simulink model "MOD5"  (R2017a)
settings: Solver=FixedStepAuto  StartTime=0.0  StopTime=10  FixedStep=1/160000  RelTol=1e-3
undefined symbols (not defined in the file): H
libraries: dspmlti4 x4
settings Model: Creator=bhannigan  LastModifiedBy=bhannigan

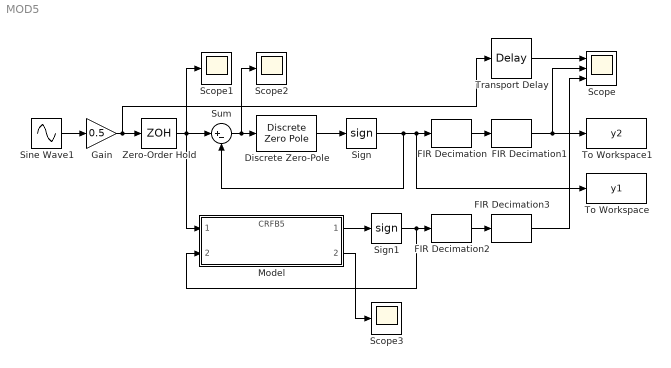
== system MOD5 ==
  Discrete Zero-Pole : DiscreteZeroPole  Zeros=H.Z{1}  Poles=H.P{1}  Gain=H.K  SampleTime=-1
  FIR Decimation{,1..3} (4 alike) : dspmlti4/FIR Decimation  FilterSource=Dialog parameters  h=fir1(31,1/64)  D=8  filtStruct=Direct form  FilterObject=FDECIM  framing=Allow multirate processing  inputOffset=0  outputBufInitCond=0  roundingMode=Floor  overflowMode=off  firstCoeffDataTypeStr=Inherit: Same word length as input  firstCoeffMin=[]  firstCoeffMax=[]  firstCoeffLastDataTypeStr=Inherit: Same word length as input  outputDataTypeStr=Inherit: Same as accumulator  outputMin=[]  outputMax=[]  outputLastDataTypeStr=Inherit: Same as accumulator
  Gain : Gain  Gain=0.5
  Model : ModelReference  ModelNameDialog=CRFB5  SimulationMode=Normal  ModelReferenceVersion=1.15
  Scope : Scope  NumInputPorts=3
  Scope1 : Scope
  Scope2 : Scope
  Scope3 : Scope
  Sign : Signum
  Sign1 : Signum
  Sine Wave1 : Sin  Frequency=2*pi*100  SampleTime=0
  Sum : Sum  Inputs=|+-
  To Workspace : ToWorkspace  VariableName=y1  SaveFormat=Timeseries  SampleTime=-1
  To Workspace1 : ToWorkspace  VariableName=y2  SaveFormat=Timeseries  SampleTime=-1
  Transport Delay : TransportDelay  DelayTime=126/160000
  Zero-Order Hold : ZeroOrderHold  SampleTime=1/160000
  wires:
  Sum/1 -> Scope2/1, Discrete Zero-Pole/1
  Discrete Zero-Pole/1 -> Sign/1
  Gain/1 -> Transport Delay/1, Zero-Order Hold/1
  Zero-Order Hold/1 -> Model/1, Sum/1, Scope1/1
  Sign/1 -> Sum/2, To Workspace/1, FIR Decimation/1
  Sine Wave1/1 -> Gain/1
  FIR Decimation/1 -> FIR Decimation1/1
  FIR Decimation1/1 -> Scope/2, To Workspace1/1
  Model/1 -> Sign1/1
  FIR Decimation3/1 -> Scope/3
  FIR Decimation2/1 -> FIR Decimation3/1
  Model/2 -> Scope3/1
  Sign1/1 -> FIR Decimation2/1, Model/2
  Transport Delay/1 -> Scope/1
